simulink model "Decoupled_System"  (R2017a)
settings: Solver=VariableStepAuto  StartTime=0.0  StopTime=35  RelTol=1e-3
values from neighbouring files (symbols this model uses):
  bm1 = 0    [OBS_CONT.m]    (also in OBS_CONT_MORE_STIFF.m)
  bm2 = 0.4402    [OBS_CONT.m]    (also in OBS_CONT_MORE_STIFF.m)
  D = zeros(1,1)    [OBS_CONT.m]
  Dm = zeros(1,1)    [OBS_CONT.m]    (also in OBS_CONT_MORE_STIFF.m)
  F = [0 1 0 0;-k/j2 -b/j2 k/j2 b/j2;0 0 0 01;k/j1 b/j1 -k/j1 -b/j1]    [OBS_CONT.m]
  Fm = [0 1 0 0;-km2/jm2 -bm2/jm2 0 0;0 0 0 1;0 0 -km1/jm1 -bm1/jm1]    [OBS_CONT.m]    (also in OBS_CONT_MORE_STIFF.m)
  G = [0;0;0;1/j1]    [OBS_CONT.m]
  Gm = [0;1/jm2;0;1/jm1]    [OBS_CONT.m]    (also in OBS_CONT_MORE_STIFF.m)
  H = [1 0 0 0]    [OBS_CONT.m]
  Hm = [1 0 0 0]*phi2    [OBS_CONT.m]    (also in OBS_CONT_MORE_STIFF.m)
  jm1 = 1.1    [OBS_CONT.m]    (also in OBS_CONT_MORE_STIFF.m)
  jm2 = 11    [OBS_CONT.m]    (also in OBS_CONT_MORE_STIFF.m)
  km1 = 0    [OBS_CONT.m]    (also in OBS_CONT_MORE_STIFF.m)
  km2 = 11.011    [OBS_CONT.m]    (also in OBS_CONT_MORE_STIFF.m)
settings Model: Creator=ASUS  LastModifiedBy=ASUS

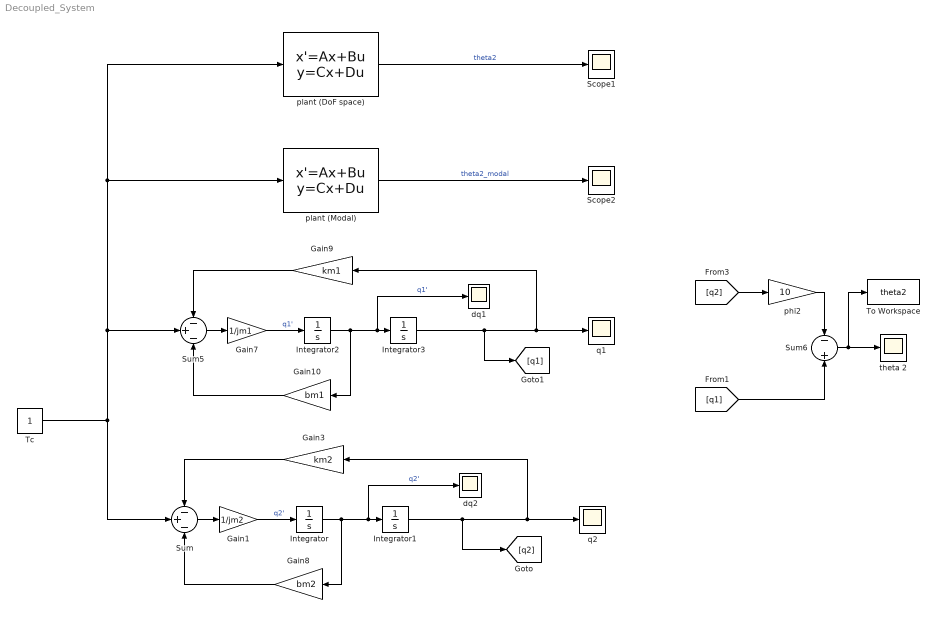
== system Decoupled_System ==
  Gain1 : Gain  Gain=1/jm2
  Gain10 : Gain  Gain=bm1
  Gain3 : Gain  Gain=km2
  Gain7 : Gain  Gain=1/jm1
  Gain8 : Gain  Gain=bm2
  Gain9 : Gain  Gain=km1
  Integrator{,1..3} (4 alike) : Integrator
  Scope1 : Scope
  Scope2 : Scope
  Sum : Sum  Inputs=-+-
  Sum5 : Sum  Inputs=-+-
  Sum6 : Sum  Inputs=-+
  Tc : Constant
  To Workspace : ToWorkspace  VariableName=theta2  SaveFormat=Timeseries  SampleTime=-1
  dq1 : Scope
  dq2 : Scope
  "phi2 " : Gain  Gain=10
  plant (DoF space) : StateSpace  A=F  B=G  C=H  D=D  X0=0
  plant (Modal) : StateSpace  A=Fm  B=Gm  C=Hm  D=Dm  X0=0
  q1 : Scope
  "q2 " : Scope
  theta 2 : Scope
  wires:
  Integrator1/1 -> [q2], Gain3/1, "q2 "/1
  Integrator2/1 -> Integrator3/1, dq1/1, Gain10/1  "q1'"
  [q1] -> Sum6/2
  plant (DoF space)/1 -> Scope1/1  "theta2"
  Sum6/1 -> To Workspace/1, theta 2/1
  Gain7/1 -> Integrator2/1  "q1'"
  Gain10/1 -> Sum5/3
  Tc/1 -> Sum5/2, plant (Modal)/1, plant (DoF space)/1, Sum/2
  Sum5/1 -> Gain7/1
  Gain3/1 -> Sum/1
  [q2] -> "phi2 "/1
  "phi2 "/1 -> Sum6/1
  Integrator/1 -> Gain8/1, dq2/1, Integrator1/1  "q2'"
  plant (Modal)/1 -> Scope2/1  "theta2_modal"
  Gain1/1 -> Integrator/1  "q2'"
  Gain8/1 -> Sum/3
  Integrator3/1 -> q1/1, Gain9/1, [q1]
  Gain9/1 -> Sum5/1
  Sum/1 -> Gain1/1
